simulink model "ldpc_decoder"  (R2025a)
settings: Solver=VariableStepAuto  StartTime=0.0  StopTime=10.0  RelTol=1e-3
libraries: whdledac x1, whdlutilities x1
settings Model: Creator=daniel  LastModifiedBy=daniel
settings OptimizationCC: BlockReduction=off  ConditionallyExecuteInputs=off

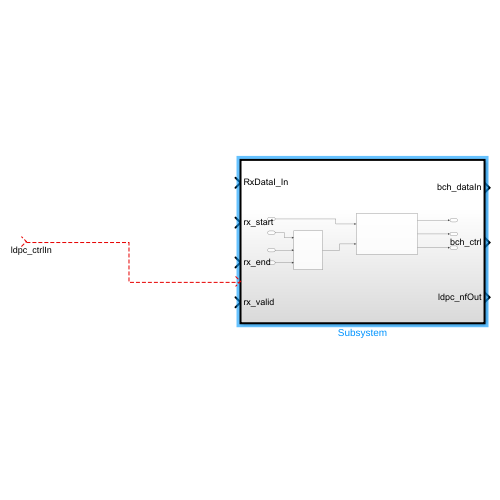
[thumbnail: Simulink's stored preview of the top-level diagram]
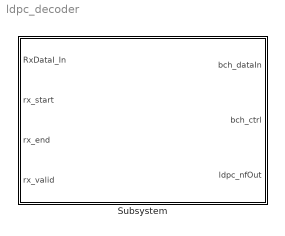
== system ldpc_decoder ==
  Subsystem : Subsystem  TreatAsAtomicUnit=on
  wires:
  ? -> ?  "ldpc_ctrlIn"

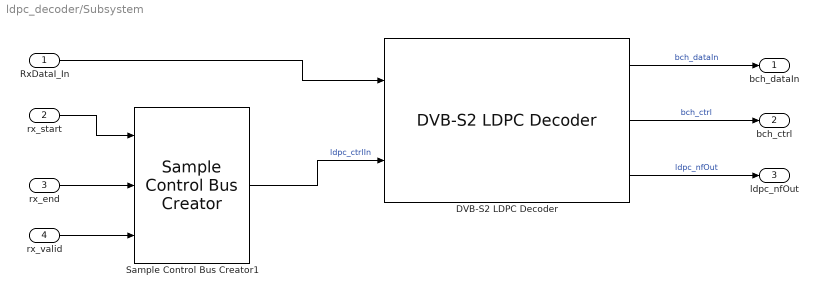
== system ldpc_decoder/Subsystem ==
  RxDataI_In : Inport  OutDataTypeStr=fixdt(1,8,4)  SampleTime=1/10e3
  rx_start : Inport  Port=2  OutDataTypeStr=boolean  SampleTime=1/10e3
  rx_end : Inport  Port=3  OutDataTypeStr=boolean  SampleTime=1/10e3
  rx_valid : Inport  Port=4  OutDataTypeStr=boolean  SampleTime=1/10e3
  DVB-S2 LDPC Decoder : whdledac/DVB-S2 LDPC Decoder  FECFrameSource=Property  FECFrame=Short  CodeRateSource=Property  CodeRateNormal=1/4  CodeRateShort=1/4  Parallelism=180  Algorithm=Min-sum  SourceScalingFactor=Property  ScalingFactor=0.75  Termination=Max  SpecifyInputs=Property  NumIterations=4  MaxNumIterations=8  ParityCheckStatus=off  SimulateUsing=Code generation
  Sample Control Bus Creator1 : whdlutilities/Sample Control Bus Creator
  bch_dataIn : Outport
  bch_ctrl : Outport  Port=2
  ldpc_nfOut : Outport  Port=3
  wires:
  DVB-S2 LDPC Decoder/1 -> bch_dataIn/1  "bch_dataIn"
  RxDataI_In/1 -> DVB-S2 LDPC Decoder/1
  DVB-S2 LDPC Decoder/2 -> bch_ctrl/1  "bch_ctrl"
  DVB-S2 LDPC Decoder/3 -> ldpc_nfOut/1  "ldpc_nfOut"
  Sample Control Bus Creator1/1 -> DVB-S2 LDPC Decoder/2  "ldpc_ctrlIn"
  rx_start/1 -> Sample Control Bus Creator1/1
  rx_end/1 -> Sample Control Bus Creator1/2
  rx_valid/1 -> Sample Control Bus Creator1/3
